simulink model "PDPWM_Three_Phase_Three_Level_Flying_Capacitor"  (R2022a)
settings: Solver=ode4  StartTime=0.0  StopTime=0.1  FixedStep=1e-5  RelTol=1e-3
libraries: spsIGBTDiodeLib x12, spsSeriesRLCBranchLib x8, simulink x6, spsVoltageMeasurementLib x4, spsCurrentMeasurementLib x3, spsGroundLib x2, spsDCVoltageSourceLib x1, spsThreePhaseVIMeasurementLib x1, spspowerguiLib x1
settings Model: Creator=nikos  LastModifiedBy=nikos

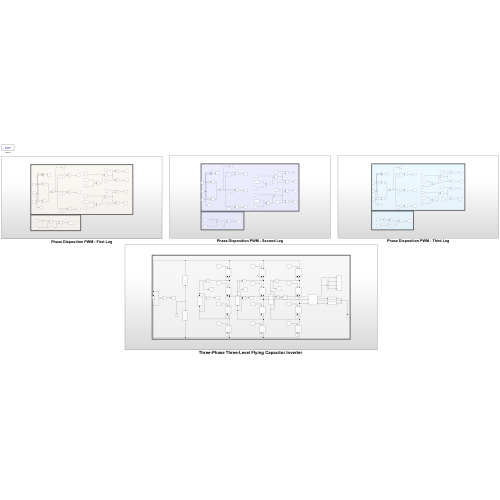
[thumbnail: Simulink's stored preview of the top-level diagram]
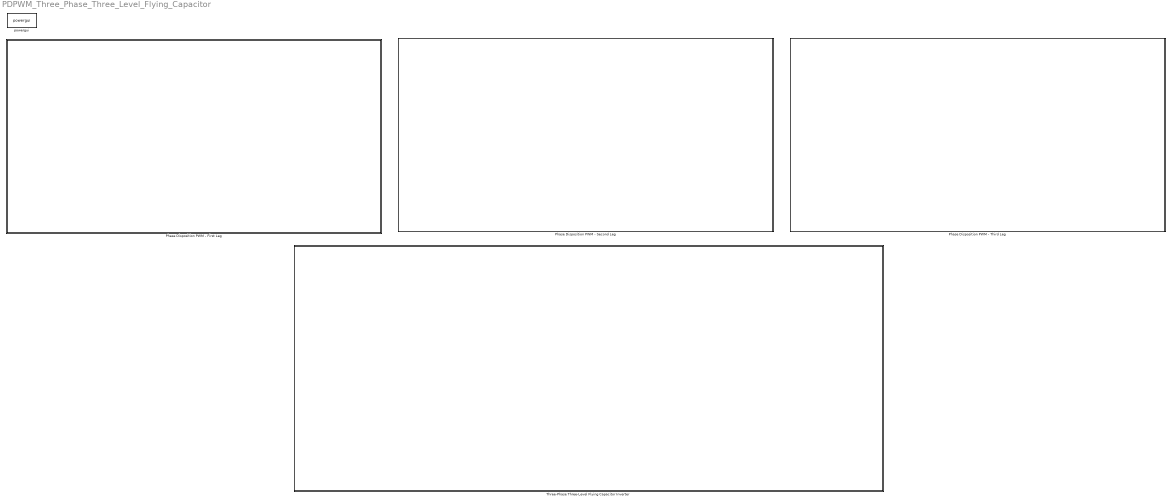
== system PDPWM_Three_Phase_Three_Level_Flying_Capacitor ==
  Phase Disposition PWM - First Leg : Subsystem
  Phase Disposition PWM - Second Leg : Subsystem
  Phase Disposition PWM - Third Leg : Subsystem
  "Three-Phase Three-Level Flying Capacitor Inverter " : Subsystem
  powergui : spspowerguiLib/powergui  Priority=1  SimulationMode=Discrete  SampleTime=1e-5  frequency=60  Iterations=50  frequencyindice=0  Pbase=100e6  ErrMax=1e-4  UnitsV=kV  UnitsW=MW  buscounter=0  FunctionMessages=off  echomessages=off  EnableUseOfTLC=off  CurrentSourceSwitches=off  DisableSnubberDevices=off  DisableRonSwitches=off  DisableVfSwitches=off  DisplayEquations=off  AutomaticDiscreteSolvers=off  SolverType=Tustin/Backward Euler (TBE)  Interpol=off  ExternalGateDelay=off  methode=off  Ts=100  x0status=blocks  SPID=on  SwTol=0  HookPort=off  NonlinearTolerance=1e-4  nMaxIteration=100  ContinueOnMaxIteration=off  RestoreLinks=warning  ResistiveCurrentMeasurement=off  Frange=[0:2:500]  Ylog=off  Xlog=on  ShowGrid=off  save=off  variable=ZData  structure=0  ZoomFFT=off  StartTime=0.0  cycles=1  DisplayStyle=1  fundamental=60  FreqAxis=off  MaxFrequency=1000  frequencyindicesteady=1  RmsSteady=1  display=off

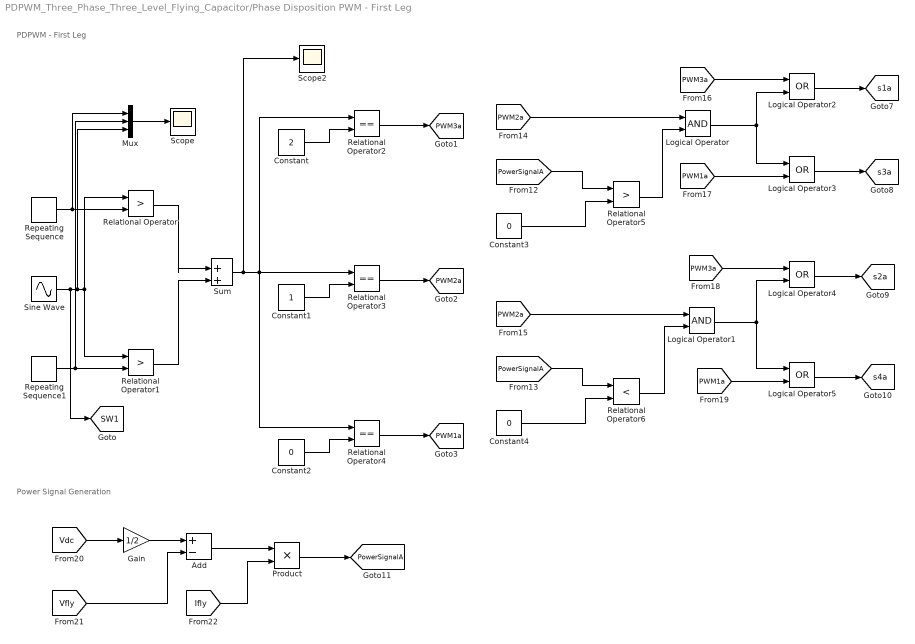
== system PDPWM_Three_Phase_Three_Level_Flying_Capacitor/Phase Disposition PWM - First Leg ==
  note: Power Signal Generation
  note: PDPWM - First Leg
  Add : Sum  Inputs=+-
  Constant : Constant  Value=2
  Constant1 : Constant
  Constant2 : Constant  Value=0
  Constant3 : Constant  Value=0
  Constant4 : Constant  Value=0
  Gain : Gain  Gain=1/2
  Logical Operator : Logic  AllPortsSameDT=off  OutDataTypeStr=boolean
  Logical Operator1 : Logic  AllPortsSameDT=off  OutDataTypeStr=boolean
  Logical Operator{2..5} (4 alike) : Logic  Operator=OR  AllPortsSameDT=off  OutDataTypeStr=boolean
  Mux : Mux  Inputs=3
  Product : Product
  Relational Operator : RelationalOperator  Operator=>  OutDataTypeStr=boolean  RndMeth=Simplest  InputSameDT=off
  Relational Operator1 : RelationalOperator  Operator=>  OutDataTypeStr=boolean  RndMeth=Simplest  InputSameDT=off
  Relational Operator2 : RelationalOperator  Operator===  OutDataTypeStr=boolean  RndMeth=Simplest  InputSameDT=off
  Relational Operator3 : RelationalOperator  Operator===  OutDataTypeStr=boolean  RndMeth=Simplest  InputSameDT=off
  Relational Operator4 : RelationalOperator  Operator===  OutDataTypeStr=boolean  RndMeth=Simplest  InputSameDT=off
  Relational Operator5 : RelationalOperator  Operator=>  OutDataTypeStr=boolean  RndMeth=Simplest  InputSameDT=off
  Relational Operator6 : RelationalOperator  Operator=<  OutDataTypeStr=boolean  RndMeth=Simplest  InputSameDT=off
  Repeating Sequence : simulink/Sources/Repeating Sequence  rep_seq_t=[0 1 2]*[1/10000]  rep_seq_y=[0 1 0]
  Repeating Sequence1 : simulink/Sources/Repeating Sequence  rep_seq_t=[0 1 2]*[1/10000]  rep_seq_y=[-1 0 -1]
  Scope : Scope
  Scope2 : Scope
  Sine Wave : Sin  Frequency=2*pi*50  SampleTime=0
  Sum : Sum  Inputs=|++
  tag scope: PWM1a=global, PWM2a=global, PWM3a=global, PowerSignalA=global, SW1=global, s1a=global, s2a=global, s3a=global, s4a=global
  wires:
  Relational Operator1/1 -> Sum/2
  Constant/1 -> Relational Operator2/2
  [Vfly] -> Add/2
  Repeating Sequence1/1 -> Relational Operator1/2, Mux/2
  Relational Operator4/1 -> [PWM1a]
  Sine Wave/1 -> [SW1], Mux/3, Relational Operator1/1, Relational Operator/1
  Repeating Sequence/1 -> Mux/1, Relational Operator/2
  Add/1 -> Product/1
  Sum/1 -> Scope2/1, Relational Operator4/1, Relational Operator2/1, Relational Operator3/1
  [Ifly] -> Product/2
  Relational Operator3/1 -> [PWM2a]
  [Vdc] -> Gain/1
  Mux/1 -> Scope/1
  Constant1/1 -> Relational Operator3/2
  Product/1 -> [PowerSignalA]
  Relational Operator/1 -> Sum/1
  Relational Operator2/1 -> [PWM3a]
  Constant2/1 -> Relational Operator4/2
  Gain/1 -> Add/1
  Logical Operator1/1 -> Logical Operator5/1, Logical Operator4/2
  Logical Operator/1 -> Logical Operator2/2, Logical Operator3/1
  Relational Operator6/1 -> Logical Operator1/2
  [PWM2a] -> Logical Operator1/1
  [PWM3a] -> Logical Operator4/1
  [PWM1a] -> Logical Operator5/2
  [PWM2a] -> Logical Operator/1
  [PowerSignalA] -> Relational Operator6/1
  Constant4/1 -> Relational Operator6/2
  [PWM1a] -> Logical Operator3/2
  Logical Operator4/1 -> [s2a]
  Relational Operator5/1 -> Logical Operator/2
  Logical Operator5/1 -> [s4a]
  Logical Operator3/1 -> [s3a]
  [PowerSignalA] -> Relational Operator5/1
  Constant3/1 -> Relational Operator5/2
  Logical Operator2/1 -> [s1a]
  [PWM3a] -> Logical Operator2/1

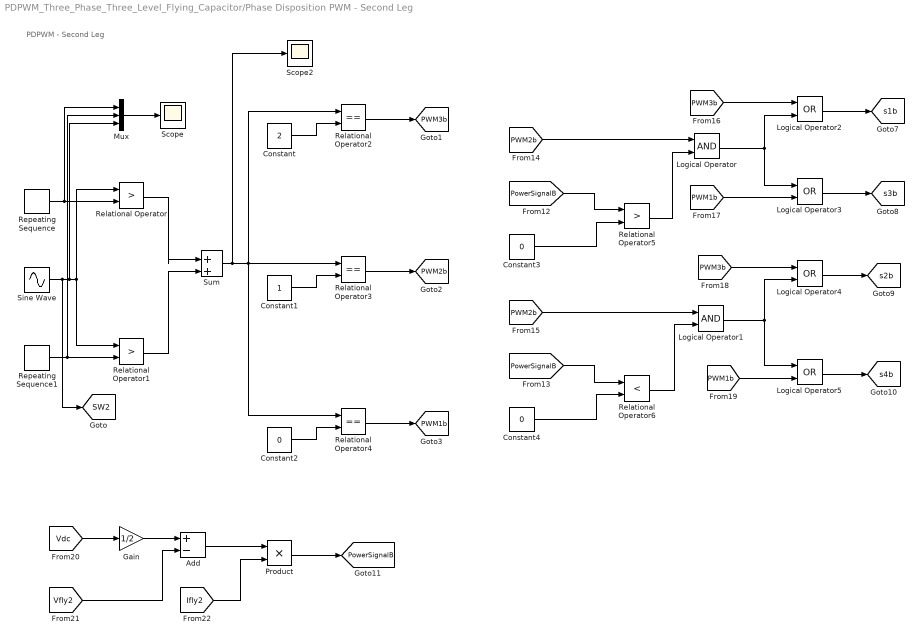
== system PDPWM_Three_Phase_Three_Level_Flying_Capacitor/Phase Disposition PWM - Second Leg ==
  note: PDPWM - Second Leg
  Add : Sum  Inputs=+-
  Constant : Constant  Value=2
  Constant1 : Constant
  Constant2 : Constant  Value=0
  Constant3 : Constant  Value=0
  Constant4 : Constant  Value=0
  Gain : Gain  Gain=1/2
  Logical Operator : Logic  AllPortsSameDT=off  OutDataTypeStr=boolean
  Logical Operator1 : Logic  AllPortsSameDT=off  OutDataTypeStr=boolean
  Logical Operator{2..5} (4 alike) : Logic  Operator=OR  AllPortsSameDT=off  OutDataTypeStr=boolean
  Mux : Mux  Inputs=3
  Product : Product
  Relational Operator : RelationalOperator  Operator=>  OutDataTypeStr=boolean  RndMeth=Simplest  InputSameDT=off
  Relational Operator1 : RelationalOperator  Operator=>  OutDataTypeStr=boolean  RndMeth=Simplest  InputSameDT=off
  Relational Operator2 : RelationalOperator  Operator===  OutDataTypeStr=boolean  RndMeth=Simplest  InputSameDT=off
  Relational Operator3 : RelationalOperator  Operator===  OutDataTypeStr=boolean  RndMeth=Simplest  InputSameDT=off
  Relational Operator4 : RelationalOperator  Operator===  OutDataTypeStr=boolean  RndMeth=Simplest  InputSameDT=off
  Relational Operator5 : RelationalOperator  Operator=>  OutDataTypeStr=boolean  RndMeth=Simplest  InputSameDT=off
  Relational Operator6 : RelationalOperator  Operator=<  OutDataTypeStr=boolean  RndMeth=Simplest  InputSameDT=off
  Repeating Sequence : simulink/Sources/Repeating Sequence  rep_seq_t=[0 1 2]*[1/10000]  rep_seq_y=[0 1 0]
  Repeating Sequence1 : simulink/Sources/Repeating Sequence  rep_seq_t=[0 1 2]*[1/10000]  rep_seq_y=[-1 0 -1]
  Scope : Scope
  Scope2 : Scope
  Sine Wave : Sin  Frequency=2*pi*50  Phase=4*pi/3  SampleTime=0
  Sum : Sum  Inputs=|++
  tag scope: PWM1b=global, PWM2b=global, PWM3b=global, PowerSignalB=global, SW2=global, s1b=global, s2b=global, s3b=global, s4b=global
  wires:
  [PWM3b] -> Logical Operator2/1
  Logical Operator2/1 -> [s1b]
  Constant3/1 -> Relational Operator5/2
  [PowerSignalB] -> Relational Operator5/1
  Logical Operator3/1 -> [s3b]
  Logical Operator5/1 -> [s4b]
  Relational Operator5/1 -> Logical Operator/2
  Logical Operator4/1 -> [s2b]
  [PWM1b] -> Logical Operator3/2
  Constant4/1 -> Relational Operator6/2
  [PowerSignalB] -> Relational Operator6/1
  [PWM2b] -> Logical Operator/1
  [PWM1b] -> Logical Operator5/2
  [PWM3b] -> Logical Operator4/1
  [PWM2b] -> Logical Operator1/1
  Relational Operator6/1 -> Logical Operator1/2
  Logical Operator/1 -> Logical Operator3/1, Logical Operator2/2
  Logical Operator1/1 -> Logical Operator4/2, Logical Operator5/1
  Gain/1 -> Add/1
  Constant2/1 -> Relational Operator4/2
  Relational Operator2/1 -> [PWM3b]
  Relational Operator/1 -> Sum/1
  Product/1 -> [PowerSignalB]
  Constant1/1 -> Relational Operator3/2
  Mux/1 -> Scope/1
  [Vdc] -> Gain/1
  Relational Operator3/1 -> [PWM2b]
  [Ifly2] -> Product/2
  Sum/1 -> Relational Operator3/1, Relational Operator2/1, Relational Operator4/1, Scope2/1
  Add/1 -> Product/1
  Repeating Sequence/1 -> Relational Operator/2, Mux/1
  Sine Wave/1 -> Relational Operator/1, Relational Operator1/1, Mux/3, [SW2]
  Relational Operator4/1 -> [PWM1b]
  Repeating Sequence1/1 -> Mux/2, Relational Operator1/2
  [Vfly2] -> Add/2
  Constant/1 -> Relational Operator2/2
  Relational Operator1/1 -> Sum/2

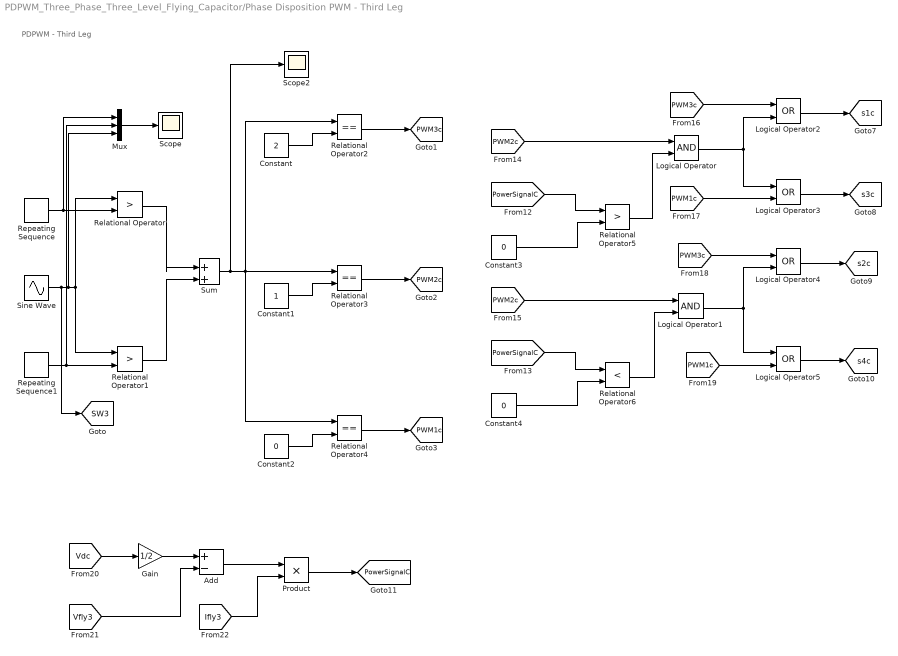
== system PDPWM_Three_Phase_Three_Level_Flying_Capacitor/Phase Disposition PWM - Third Leg ==
  note: PDPWM - Third Leg
  Add : Sum  Inputs=+-
  Constant : Constant  Value=2
  Constant1 : Constant
  Constant2 : Constant  Value=0
  Constant3 : Constant  Value=0
  Constant4 : Constant  Value=0
  Gain : Gain  Gain=1/2
  Logical Operator : Logic  AllPortsSameDT=off  OutDataTypeStr=boolean
  Logical Operator1 : Logic  AllPortsSameDT=off  OutDataTypeStr=boolean
  Logical Operator{2..5} (4 alike) : Logic  Operator=OR  AllPortsSameDT=off  OutDataTypeStr=boolean
  Mux : Mux  Inputs=3
  Product : Product
  Relational Operator : RelationalOperator  Operator=>  OutDataTypeStr=boolean  RndMeth=Simplest  InputSameDT=off
  Relational Operator1 : RelationalOperator  Operator=>  OutDataTypeStr=boolean  RndMeth=Simplest  InputSameDT=off
  Relational Operator2 : RelationalOperator  Operator===  OutDataTypeStr=boolean  RndMeth=Simplest  InputSameDT=off
  Relational Operator3 : RelationalOperator  Operator===  OutDataTypeStr=boolean  RndMeth=Simplest  InputSameDT=off
  Relational Operator4 : RelationalOperator  Operator===  OutDataTypeStr=boolean  RndMeth=Simplest  InputSameDT=off
  Relational Operator5 : RelationalOperator  Operator=>  OutDataTypeStr=boolean  RndMeth=Simplest  InputSameDT=off
  Relational Operator6 : RelationalOperator  Operator=<  OutDataTypeStr=boolean  RndMeth=Simplest  InputSameDT=off
  Repeating Sequence : simulink/Sources/Repeating Sequence  rep_seq_t=[0 1 2]*[1/10000]  rep_seq_y=[0 1 0]
  Repeating Sequence1 : simulink/Sources/Repeating Sequence  rep_seq_t=[0 1 2]*[1/10000]  rep_seq_y=[-1 0 -1]
  Scope : Scope
  Scope2 : Scope
  Sine Wave : Sin  Frequency=2*pi*50  Phase=2*pi/3  SampleTime=0
  Sum : Sum  Inputs=|++
  tag scope: PWM1c=global, PWM2c=global, PWM3c=global, PowerSignalC=global, SW3=global, s1c=global, s2c=global, s3c=global, s4c=global
  wires:
  Relational Operator1/1 -> Sum/2
  Constant/1 -> Relational Operator2/2
  [Vfly3] -> Add/2
  Repeating Sequence1/1 -> Relational Operator1/2, Mux/2
  Relational Operator4/1 -> [PWM1c]
  Sine Wave/1 -> [SW3], Mux/3, Relational Operator1/1, Relational Operator/1
  Repeating Sequence/1 -> Mux/1, Relational Operator/2
  Add/1 -> Product/1
  Sum/1 -> Scope2/1, Relational Operator4/1, Relational Operator2/1, Relational Operator3/1
  [Ifly3] -> Product/2
  Relational Operator3/1 -> [PWM2c]
  [Vdc] -> Gain/1
  Mux/1 -> Scope/1
  Constant1/1 -> Relational Operator3/2
  Product/1 -> [PowerSignalC]
  Relational Operator/1 -> Sum/1
  Relational Operator2/1 -> [PWM3c]
  Constant2/1 -> Relational Operator4/2
  Gain/1 -> Add/1
  Logical Operator1/1 -> Logical Operator5/1, Logical Operator4/2
  Logical Operator/1 -> Logical Operator2/2, Logical Operator3/1
  Relational Operator6/1 -> Logical Operator1/2
  [PWM2c] -> Logical Operator1/1
  [PWM3c] -> Logical Operator4/1
  [PWM1c] -> Logical Operator5/2
  [PWM2c] -> Logical Operator/1
  [PowerSignalC] -> Relational Operator6/1
  Constant4/1 -> Relational Operator6/2
  [PWM1c] -> Logical Operator3/2
  Logical Operator4/1 -> [s2c]
  Relational Operator5/1 -> Logical Operator/2
  Logical Operator5/1 -> [s4c]
  Logical Operator3/1 -> [s3c]
  [PowerSignalC] -> Relational Operator5/1
  Constant3/1 -> Relational Operator5/2
  Logical Operator2/1 -> [s1c]
  [PWM3c] -> Logical Operator2/1

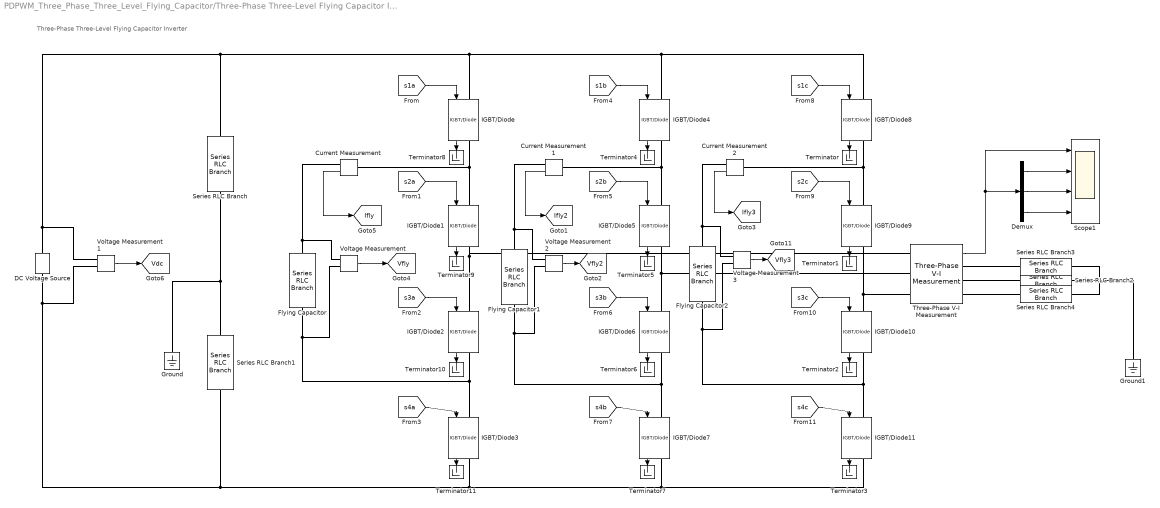
== system PDPWM_Three_Phase_Three_Level_Flying_Capacitor/Three-Phase Three-Level Flying Capacitor Inverter  ==
  note: Three-Phase Three-Level Flying Capacitor Inverter
  Current Measurement : spsCurrentMeasurementLib/Current Measurement  PhasorSimulation=off  OutputType=Complex  PSBequivalent=0
  Current Measurement1 : spsCurrentMeasurementLib/Current Measurement  PhasorSimulation=off  OutputType=Complex  PSBequivalent=0
  Current Measurement2 : spsCurrentMeasurementLib/Current Measurement  PhasorSimulation=off  OutputType=Complex  PSBequivalent=0
  DC Voltage Source : spsDCVoltageSourceLib/DC Voltage Source  Amplitude=100  Measurements=None
  Demux : Demux  Outputs=3
  Flying Capacitor : spsSeriesRLCBranchLib/Series RLC Branch  LConnTagsString=__new0  RConnTagsString=__new0  BranchType=RC  Resistance=0.01  Inductance=1e-3  SetiL0=off  InitialCurrent=0  Capacitance=4.7e-3  Setx0=off  InitialVoltage=0  Measurements=None
  Flying Capacitor1 : spsSeriesRLCBranchLib/Series RLC Branch  LConnTagsString=__new0  RConnTagsString=__new0  BranchType=RC  Resistance=0.01  Inductance=1e-3  SetiL0=off  InitialCurrent=0  Capacitance=4.7e-3  Setx0=off  InitialVoltage=0  Measurements=None
  Flying Capacitor2 : spsSeriesRLCBranchLib/Series RLC Branch  LConnTagsString=__new0  RConnTagsString=__new0  BranchType=RC  Resistance=0.01  Inductance=1e-3  SetiL0=off  InitialCurrent=0  Capacitance=4.7e-3  Setx0=off  InitialVoltage=0  Measurements=None
  Ground : spsGroundLib/Ground  LConnTagsString=a
  Ground1 : spsGroundLib/Ground  LConnTagsString=a
  IGBT/Diode{,1..11} (12 alike) : spsIGBTDiodeLib/IGBT//Diode  Ron=1e-3  Rs=1e5  Cs=inf  Measurements=on
  Scope1 : Scope  NumInputPorts=4
  Series RLC Branch : spsSeriesRLCBranchLib/Series RLC Branch  LConnTagsString=__new0  RConnTagsString=__new0  BranchType=RC  Resistance=0.01  Inductance=1e-3  SetiL0=off  InitialCurrent=0  Capacitance=4.7e-3  Setx0=off  InitialVoltage=0  Measurements=None
  Series RLC Branch1 : spsSeriesRLCBranchLib/Series RLC Branch  LConnTagsString=__new0  RConnTagsString=__new0  BranchType=RC  Resistance=0.01  Inductance=1e-3  SetiL0=off  InitialCurrent=0  Capacitance=4.7e-3  Setx0=off  InitialVoltage=0  Measurements=None
  Series RLC Branch2 : spsSeriesRLCBranchLib/Series RLC Branch  LConnTagsString=__new0  RConnTagsString=__new0  BranchType=R  Resistance=100  Inductance=1e-3  SetiL0=off  InitialCurrent=0  Capacitance=1e-6  Setx0=off  InitialVoltage=0  Measurements=None
  Series RLC Branch3 : spsSeriesRLCBranchLib/Series RLC Branch  LConnTagsString=__new0  RConnTagsString=__new0  BranchType=R  Resistance=100  Inductance=1e-3  SetiL0=off  InitialCurrent=0  Capacitance=1e-6  Setx0=off  InitialVoltage=0  Measurements=None
  Series RLC Branch4 : spsSeriesRLCBranchLib/Series RLC Branch  LConnTagsString=__new0  RConnTagsString=__new0  BranchType=R  Resistance=100  Inductance=1e-3  SetiL0=off  InitialCurrent=0  Capacitance=1e-6  Setx0=off  InitialVoltage=0  Measurements=None
  Terminator{,1..11} (12 alike) : Terminator
  Three-Phase V-I Measurement : spsThreePhaseVIMeasurementLib/Three-Phase V-I Measurement  VoltageMeasurement=phase-to-ground  SetLabelV=off  LabelV=Vabc  Vpu=off  VpuLL=off  CurrentMeasurement=no  SetLabelI=off  LabelI=Iabc  Ipu=off  Pbase=100e6  Vbase=500e3  OutputType=Complex  PhasorSimulation=off  PSBequivalent=0
  Voltage Measurement{,1..3} (4 alike) : spsVoltageMeasurementLib/Voltage Measurement  PhasorSimulation=off  OutputType=Complex  PSBequivalent=0
  tag scope: Ifly2=global, Ifly3=global, Ifly=global, Vdc=global, Vfly2=global, Vfly3=global, Vfly=global
  wires:
  Voltage Measurement/1 -> [Vfly]
  Voltage Measurement3/1 -> [Vfly3]
  Demux/1 -> Scope1/2
  [s4b] -> IGBT/Diode7/1
  IGBT/Diode/1 -> Terminator8/1
  IGBT/Diode1/1 -> Terminator9/1
  Current Measurement1/1 -> [Ifly2]
  IGBT/Diode9/1 -> Terminator1/1
  [s2b] -> IGBT/Diode5/1
  [s1c] -> IGBT/Diode8/1
  IGBT/Diode10/1 -> Terminator2/1
  IGBT/Diode5/1 -> Terminator5/1
  [s1a] -> IGBT/Diode/1
  IGBT/Diode7/1 -> Terminator7/1
  IGBT/Diode6/1 -> Terminator6/1
  [s4c] -> IGBT/Diode11/1
  IGBT/Diode4/1 -> Terminator4/1
  IGBT/Diode8/1 -> Terminator/1
  [s2c] -> IGBT/Diode9/1
  [s3c] -> IGBT/Diode10/1
  IGBT/Diode2/1 -> Terminator10/1
  [s3b] -> IGBT/Diode6/1
  [s4a] -> IGBT/Diode3/1
  [s2a] -> IGBT/Diode1/1
  Voltage Measurement2/1 -> [Vfly2]
  IGBT/Diode11/1 -> Terminator3/1
  Demux/2 -> Scope1/3
  IGBT/Diode3/1 -> Terminator11/1
  Current Measurement/1 -> [Ifly]
  Three-Phase V-I Measurement/1 -> Demux/1, Scope1/1
  Demux/3 -> Scope1/4
  [s3a] -> IGBT/Diode2/1
  [s1b] -> IGBT/Diode4/1
  Voltage Measurement1/1 -> [Vdc]
  Current Measurement2/1 -> [Ifly3]
  connections:
  IGBT/Diode2/RConn1 -- IGBT/Diode3/LConn1 -- Voltage Measurement/LConn2 -- Flying Capacitor/RConn1
  Three-Phase V-I Measurement/RConn1 -- Series RLC Branch3/RConn1
  IGBT/Diode9/RConn1 -- Three-Phase V-I Measurement/LConn3 -- IGBT/Diode10/LConn1
  Series RLC Branch2/LConn1 -- Ground1/LConn1 -- Series RLC Branch4/LConn1 -- Series RLC Branch3/LConn1
  IGBT/Diode/RConn1 -- Current Measurement/LConn1 -- IGBT/Diode1/LConn1
  Series RLC Branch1/LConn1 -- Ground/LConn1 -- Series RLC Branch/RConn1
  Voltage Measurement3/LConn2 -- IGBT/Diode10/RConn1 -- IGBT/Diode11/LConn1 -- Flying Capacitor2/RConn1
  IGBT/Diode11/RConn1 -- IGBT/Diode7/RConn1 -- Voltage Measurement1/LConn2 -- DC Voltage Source/LConn1 -- Series RLC Branch1/RConn1 -- IGBT/Diode3/RConn1
  Three-Phase V-I Measurement/RConn3 -- Series RLC Branch4/RConn1
  IGBT/Diode8/LConn1 -- IGBT/Diode4/LConn1 -- DC Voltage Source/RConn1 -- Voltage Measurement1/LConn1 -- Series RLC Branch/LConn1 -- IGBT/Diode/LConn1
  Flying Capacitor/LConn1 -- Current Measurement/RConn1 -- Voltage Measurement/LConn1
  IGBT/Diode4/RConn1 -- Current Measurement1/LConn1 -- IGBT/Diode5/LConn1
  IGBT/Diode5/RConn1 -- Three-Phase V-I Measurement/LConn2 -- IGBT/Diode6/LConn1
  Three-Phase V-I Measurement/RConn2 -- Series RLC Branch2/RConn1
  IGBT/Diode8/RConn1 -- Current Measurement2/LConn1 -- IGBT/Diode9/LConn1
  IGBT/Diode1/RConn1 -- IGBT/Diode2/LConn1 -- Three-Phase V-I Measurement/LConn1
  IGBT/Diode6/RConn1 -- IGBT/Diode7/LConn1 -- Voltage Measurement2/LConn2 -- Flying Capacitor1/RConn1
  Current Measurement2/RConn1 -- Flying Capacitor2/LConn1 -- Voltage Measurement3/LConn1
  Current Measurement1/RConn1 -- Voltage Measurement2/LConn1 -- Flying Capacitor1/LConn1
